simulink model "uz_debug_switch_measurements"  (R2021a)
settings: Solver=FixedStepDiscrete  StartTime=0.0  StopTime=10.0  RelTol=1e-3
settings Model: DataTypeOverride=Off  Creator=micha  LastModifiedBy=micha
settings SolverCC: AlgebraicLoopSolver=TrustRegion
settings DataIOCC: LimitDataPoints=on  SaveOutput=off  SaveTime=off
settings OptimizationCC: BlockReduction=off  ConditionallyExecuteInputs=off  DefaultParameterBehavior=Inlined  LifeSpan=inf
settings DebuggingCC: AlgebraicLoopMsg=error  SingleTaskRateTransMsg=error  AllowSymbolicDim=off  StrictBusMsg=ErrorOnBusTreatedAsVector  SFUnexpectedBacktrackingDiag=warning  SFNoUnconditionalDefaultTransitionDiag=warning  SFExecutionAtInitializationDiag=none  SFMachineParentedDataDiag=warning  ArithmeticOperatorsInVariantConditions=warning
settings HardwareCC: ProdBitPerPointer=32  ProdBitPerSizeT=32  ProdBitPerPtrDiffT=32  ProdLargestAtomicFloat=None  ProdIntDivRoundTo=Undefined  ProdEndianess=Unspecified  ProdWordSize=32  ProdHWDeviceType=ASIC/FPGA->ASIC/FPGA  ProdEqTarget=off
settings SFSimCC: SimUseLocalCustomCode=off  CustomCodeUndefinedFunction=UseInterfaceOnly
settings RTWCC: RTWUseLocalCustomCode=off
settings CodeAppCC: StateflowObjectComments=on
settings GRTTargetCC: TargetLangStandard=C89/C90 (ANSI)
settings ConfigComp: CovScope=ReferencedModels  CovMetricSettings=dw  CovSaveCumulativeToWorkspaceVar=on  CovSaveSingleToWorkspaceVar=on  CovExternalEMLEnable=off  CovSFcnEnable=off

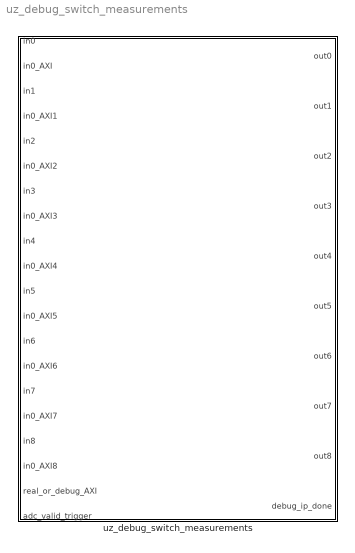
== system uz_debug_switch_measurements ==
  uz_debug_switch_measurements : Subsystem

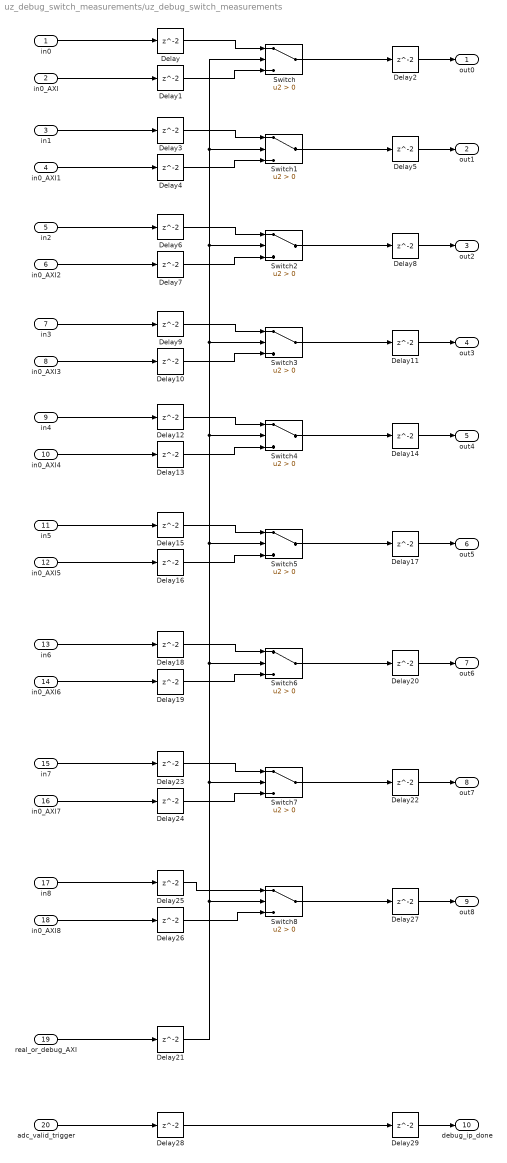
== system uz_debug_switch_measurements/uz_debug_switch_measurements ==
  in0 : Inport
  in0_AXI : Inport  Port=2
  in1 : Inport  Port=3
  in0_AXI1 : Inport  Port=4
  in2 : Inport  Port=5
  in0_AXI2 : Inport  Port=6
  in3 : Inport  Port=7
  in0_AXI3 : Inport  Port=8
  in4 : Inport  Port=9
  in0_AXI4 : Inport  Port=10
  in5 : Inport  Port=11
  in0_AXI5 : Inport  Port=12
  in6 : Inport  Port=13
  in0_AXI6 : Inport  Port=14
  in7 : Inport  Port=15
  in0_AXI7 : Inport  Port=16
  in8 : Inport  Port=17
  in0_AXI8 : Inport  Port=18
  real_or_debug_AXI : Inport  Port=19
  adc_valid_trigger : Inport  Port=20
  Delay{,1..29} (30 alike) : Delay
  Switch{,1..8} (9 alike) : Switch  Criteria=u2 > Threshold
  out0 : Outport  VectorParamsAs1DForOutWhenUnconnected=off
  out1 : Outport  Port=2  VectorParamsAs1DForOutWhenUnconnected=off
  out2 : Outport  Port=3  VectorParamsAs1DForOutWhenUnconnected=off
  out3 : Outport  Port=4  VectorParamsAs1DForOutWhenUnconnected=off
  out4 : Outport  Port=5  VectorParamsAs1DForOutWhenUnconnected=off
  out5 : Outport  Port=6  VectorParamsAs1DForOutWhenUnconnected=off
  out6 : Outport  Port=7  VectorParamsAs1DForOutWhenUnconnected=off
  out7 : Outport  Port=8  VectorParamsAs1DForOutWhenUnconnected=off
  out8 : Outport  Port=9  VectorParamsAs1DForOutWhenUnconnected=off
  debug_ip_done : Outport  Port=10  VectorParamsAs1DForOutWhenUnconnected=off
  wires:
  in0/1 -> Delay/1
  in0_AXI/1 -> Delay1/1
  Delay/1 -> Switch/1
  Delay1/1 -> Switch/3
  Switch/1 -> Delay2/1
  Delay2/1 -> out0/1
  in0_AXI1/1 -> Delay4/1
  Delay5/1 -> out1/1
  in1/1 -> Delay3/1
  Delay4/1 -> Switch1/3
  Delay3/1 -> Switch1/1
  Switch1/1 -> Delay5/1
  in0_AXI2/1 -> Delay7/1
  Delay8/1 -> out2/1
  in2/1 -> Delay6/1
  Delay7/1 -> Switch2/3
  Delay6/1 -> Switch2/1
  Switch2/1 -> Delay8/1
  in0_AXI3/1 -> Delay10/1
  Delay11/1 -> out3/1
  in3/1 -> Delay9/1
  Delay10/1 -> Switch3/3
  Delay9/1 -> Switch3/1
  Switch3/1 -> Delay11/1
  in0_AXI4/1 -> Delay13/1
  Delay14/1 -> out4/1
  in4/1 -> Delay12/1
  Delay13/1 -> Switch4/3
  Delay12/1 -> Switch4/1
  Switch4/1 -> Delay14/1
  in0_AXI5/1 -> Delay16/1
  Delay17/1 -> out5/1
  in5/1 -> Delay15/1
  Delay16/1 -> Switch5/3
  Delay15/1 -> Switch5/1
  Switch5/1 -> Delay17/1
  in0_AXI6/1 -> Delay19/1
  Delay20/1 -> out6/1
  in6/1 -> Delay18/1
  Delay19/1 -> Switch6/3
  Delay18/1 -> Switch6/1
  Switch6/1 -> Delay20/1
  real_or_debug_AXI/1 -> Delay21/1
  Delay22/1 -> out7/1
  Delay23/1 -> Switch7/1
  Delay21/1 -> Switch8/2, Switch7/2, Switch6/2, Switch5/2, Switch4/2, Switch3/2, Switch2/2, Switch/2, Switch1/2
  Delay24/1 -> Switch7/3
  Switch7/1 -> Delay22/1
  in0_AXI7/1 -> Delay24/1
  in7/1 -> Delay23/1
  in8/1 -> Delay25/1
  in0_AXI8/1 -> Delay26/1
  Switch8/1 -> Delay27/1
  Delay27/1 -> out8/1
  Delay25/1 -> Switch8/1
  Delay26/1 -> Switch8/3
  adc_valid_trigger/1 -> Delay28/1
  Delay29/1 -> debug_ip_done/1
  Delay28/1 -> Delay29/1
